simulink model "fault_lib"  (R2018b)
settings: Solver=VariableStepAuto  StartTime=0.0  StopTime=10.0  RelTol=1e-3
undefined symbols (not defined in the file): fswParams
libraries: simulink x9
settings Model: Creator=Nick's PC  LastModifiedBy=Nick's PC

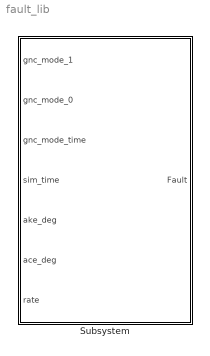
== system fault_lib ==
  Subsystem : Subsystem

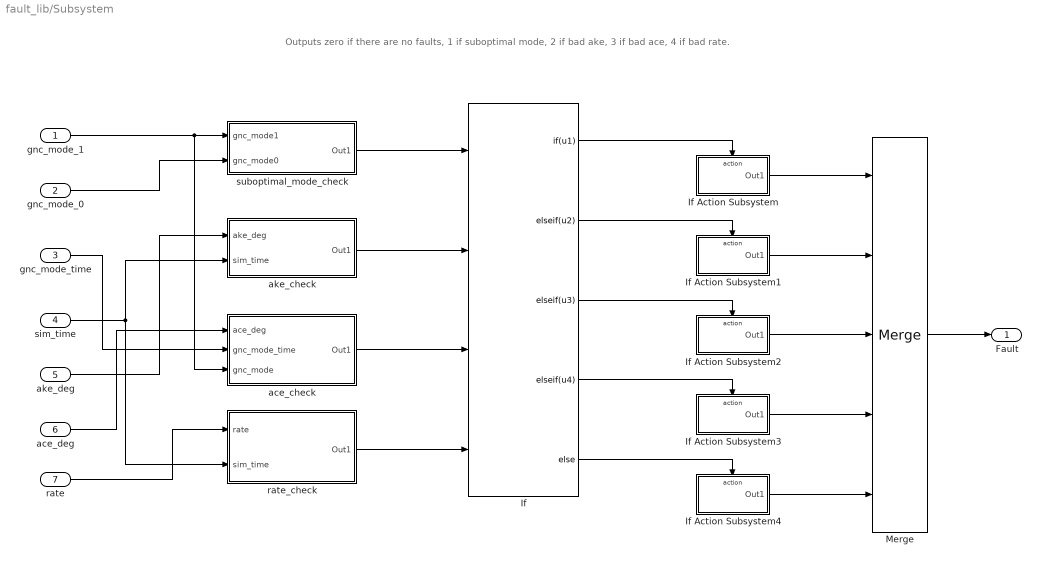
== system fault_lib/Subsystem ==
  note: Outputs zero if there are no faults, 1 if suboptimal mode, 2 if bad ake, 3 if bad ace, 4 if bad rate.
  gnc_mode_1 : Inport
  gnc_mode_0 : Inport  Port=2
  gnc_mode_time : Inport  Port=3
  sim_time : Inport  Port=4
  ake_deg : Inport  Port=5
  ace_deg : Inport  Port=6
  rate : Inport  Port=7
  If : If  NumInputs=4  IfExpression=u1  ElseIfExpressions=u2, u3, u4
  If Action Subsystem : Subsystem  TreatAsAtomicUnit=on
  If Action Subsystem1 : Subsystem  TreatAsAtomicUnit=on
  If Action Subsystem2 : Subsystem  TreatAsAtomicUnit=on
  If Action Subsystem3 : Subsystem  TreatAsAtomicUnit=on
  If Action Subsystem4 : Subsystem  TreatAsAtomicUnit=on
  Merge : Merge  Inputs=5
  ace_check : Subsystem
  ake_check : Subsystem
  rate_check : Subsystem
  suboptimal_mode_check : Subsystem
  Fault : Outport
  wires:
  gnc_mode_1/1 -> ace_check/3(gnc_mode), suboptimal_mode_check/1(gnc_mode1)
  If/1 -> If Action Subsystem/Action
  If/2 -> If Action Subsystem1/Action
  If/3 -> If Action Subsystem2/Action
  If/4 -> If Action Subsystem3/Action
  If/5 -> If Action Subsystem4/Action
  suboptimal_mode_check/1(Out1) -> If/1
  ake_check/1(Out1) -> If/2
  ace_check/1(Out1) -> If/3
  rate_check/1(Out1) -> If/4
  gnc_mode_0/1 -> suboptimal_mode_check/2(gnc_mode0)
  sim_time/1 -> ake_check/2(sim_time), rate_check/2(sim_time)
  ace_deg/1 -> ace_check/1(ace_deg)
  gnc_mode_time/1 -> ace_check/2(gnc_mode_time)
  ake_deg/1 -> ake_check/1(ake_deg)
  rate/1 -> rate_check/1(rate)
  If Action Subsystem/1(Out1) -> Merge/1
  If Action Subsystem1/1(Out1) -> Merge/2
  If Action Subsystem2/1(Out1) -> Merge/3
  If Action Subsystem3/1(Out1) -> Merge/4
  If Action Subsystem4/1(Out1) -> Merge/5
  Merge/1 -> Fault/1

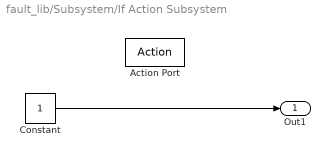
== system fault_lib/Subsystem/If Action Subsystem ==
  Action Port : ActionPort  ActionType=then
  Constant : Constant
  Out1 : Outport
  wires:
  Constant/1 -> Out1/1

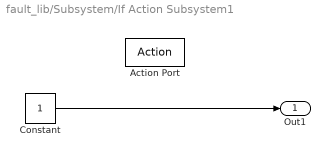
== system fault_lib/Subsystem/If Action Subsystem1 ==
  Action Port : ActionPort  ActionType=elseif
  Constant : Constant
  Out1 : Outport
  wires:
  Constant/1 -> Out1/1

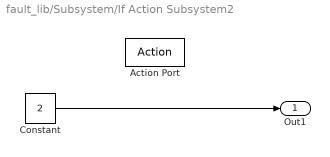
== system fault_lib/Subsystem/If Action Subsystem2 ==
  Action Port : ActionPort  ActionType=elseif
  Constant : Constant  Value=2
  Out1 : Outport
  wires:
  Constant/1 -> Out1/1

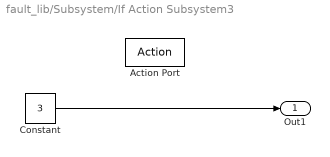
== system fault_lib/Subsystem/If Action Subsystem3 ==
  Action Port : ActionPort  ActionType=elseif
  Constant : Constant  Value=3
  Out1 : Outport
  wires:
  Constant/1 -> Out1/1

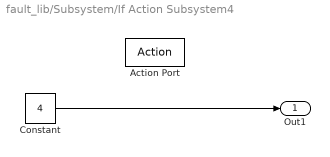
== system fault_lib/Subsystem/If Action Subsystem4 ==
  Action Port : ActionPort  ActionType=else
  Constant : Constant  Value=4
  Out1 : Outport
  wires:
  Constant/1 -> Out1/1

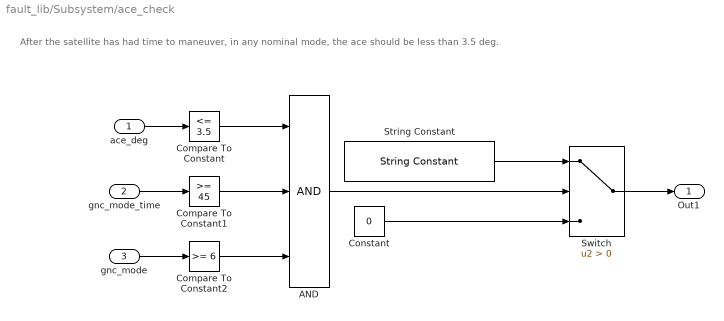
== system fault_lib/Subsystem/ace_check ==
  note: After the satellite has had time to maneuver, in any nominal mode, the ace should be less than 3.5 deg.
  ace_deg : Inport
  gnc_mode_time : Inport  Port=2
  gnc_mode : Inport  Port=3
  AND : Logic  Inputs=3  IconShape=distinctive  AllPortsSameDT=off  OutDataTypeStr=boolean
  Compare To Constant : simulink/Logic and Bit Operations/Compare To Constant  relop=<=  const=3.5  OutDataTypeStr=boolean
  Compare To Constant1 : simulink/Logic and Bit Operations/Compare To Constant  relop=>=  const=45  OutDataTypeStr=boolean
  Compare To Constant2 : simulink/Logic and Bit Operations/Compare To Constant  relop=>=  const=6  OutDataTypeStr=boolean
  Constant : Constant  Value=0  OutDataTypeStr=uint8
  String Constant : StringConstant  String="\"ACE Requirement Exceeded\""
  Switch : Switch  Criteria=u2 > Threshold
  Out1 : Outport
  wires:
  ace_deg/1 -> Compare To Constant/1
  Compare To Constant/1 -> AND/1
  gnc_mode_time/1 -> Compare To Constant1/1
  Compare To Constant1/1 -> AND/2
  gnc_mode/1 -> Compare To Constant2/1
  Compare To Constant2/1 -> AND/3
  AND/1 -> Switch/2
  Constant/1 -> Switch/3
  Switch/1 -> Out1/1
  String Constant/1 -> Switch/1

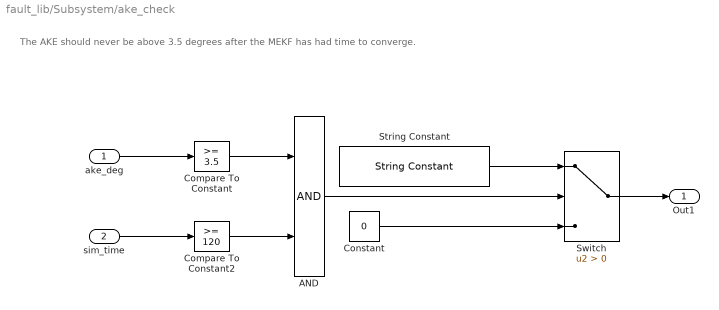
== system fault_lib/Subsystem/ake_check ==
  note: The AKE should never be above 3.5 degrees after the MEKF has had time to converge.
  ake_deg : Inport
  sim_time : Inport  Port=2
  AND : Logic  IconShape=distinctive  AllPortsSameDT=off  OutDataTypeStr=boolean
  Compare To Constant : simulink/Logic and Bit Operations/Compare To Constant  relop=>=  const=3.5  OutDataTypeStr=boolean
  Compare To Constant2 : simulink/Logic and Bit Operations/Compare To Constant  relop=>=  const=120  OutDataTypeStr=boolean
  Constant : Constant  Value=0  OutDataTypeStr=uint8
  String Constant : StringConstant  String="\"AKE Requirement Exceeded\""
  Switch : Switch  Criteria=u2 > Threshold
  Out1 : Outport
  wires:
  ake_deg/1 -> Compare To Constant/1
  Compare To Constant/1 -> AND/1
  sim_time/1 -> Compare To Constant2/1
  Compare To Constant2/1 -> AND/2
  AND/1 -> Switch/2
  Constant/1 -> Switch/3
  Switch/1 -> Out1/1
  String Constant/1 -> Switch/1

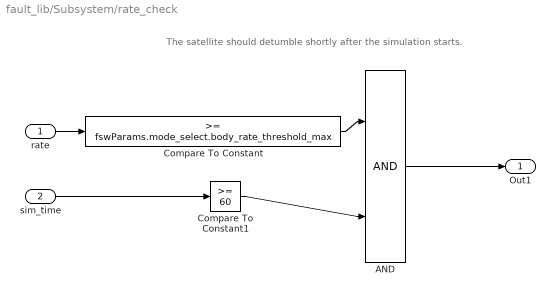
== system fault_lib/Subsystem/rate_check ==
  note: The satellite should detumble shortly after the simulation starts.
  rate : Inport
  sim_time : Inport  Port=2
  AND : Logic  IconShape=distinctive  AllPortsSameDT=off  OutDataTypeStr=boolean
  Compare To Constant : simulink/Logic and Bit Operations/Compare To Constant  relop=>=  const=fswParams.mode_select.body_rate_threshold_max  OutDataTypeStr=boolean
  Compare To Constant1 : simulink/Logic and Bit Operations/Compare To Constant  relop=>=  const=60  OutDataTypeStr=boolean
  Out1 : Outport
  wires:
  rate/1 -> Compare To Constant/1
  Compare To Constant/1 -> AND/1
  sim_time/1 -> Compare To Constant1/1
  Compare To Constant1/1 -> AND/2
  AND/1 -> Out1/1

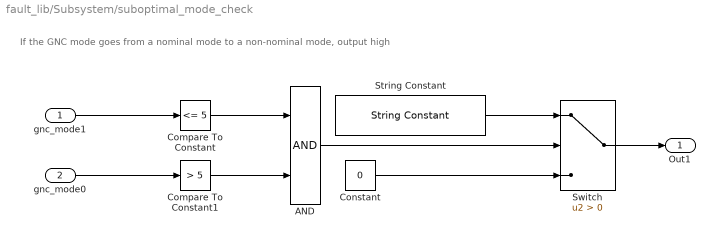
== system fault_lib/Subsystem/suboptimal_mode_check ==
  note: If the GNC mode goes from a nominal mode to a non-nominal mode, output high
  gnc_mode1 : Inport
  gnc_mode0 : Inport  Port=2
  AND : Logic  IconShape=distinctive  AllPortsSameDT=off  OutDataTypeStr=boolean
  Compare To Constant : simulink/Logic and Bit Operations/Compare To Constant  relop=<=  const=5  OutDataTypeStr=boolean
  Compare To Constant1 : simulink/Logic and Bit Operations/Compare To Constant  relop=>  const=5  OutDataTypeStr=boolean
  Constant : Constant  Value=0  OutDataTypeStr=uint8
  String Constant : StringConstant  String="\"Suboptimal GNC Mode\""
  Switch : Switch  Criteria=u2 > Threshold
  Out1 : Outport
  wires:
  gnc_mode1/1 -> Compare To Constant/1
  Compare To Constant/1 -> AND/1
  gnc_mode0/1 -> Compare To Constant1/1
  Compare To Constant1/1 -> AND/2
  AND/1 -> Switch/2
  Constant/1 -> Switch/3
  Switch/1 -> Out1/1
  String Constant/1 -> Switch/1
